simulink model "motor_ctrl"  (R2021a)
settings: configuration reference "f2_ctrl_config" (kept outside this file)
settings Model: DataDictionary=motor_data.sldd  Creator=Litao  LastModifiedBy=Litao
settings ConfigSetRef: SourceName=f2_ctrl_config

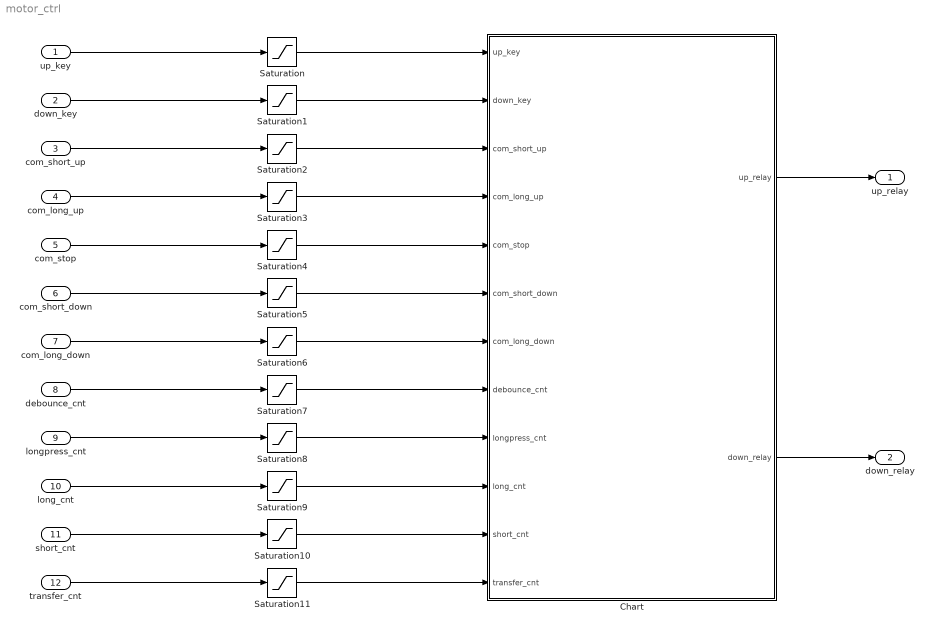
== system motor_ctrl ==
  up_key : Inport  OutDataTypeStr=int16
  down_key : Inport  Port=2  OutDataTypeStr=int16
  com_short_up : Inport  Port=3  OutDataTypeStr=int16
  com_long_up : Inport  Port=4  OutDataTypeStr=int16
  com_stop : Inport  Port=5  OutDataTypeStr=int16
  com_short_down : Inport  Port=6  OutDataTypeStr=int16
  com_long_down : Inport  Port=7  OutDataTypeStr=int16
  debounce_cnt : Inport  Port=8  OutDataTypeStr=int16
  longpress_cnt : Inport  Port=9  OutDataTypeStr=int16
  long_cnt : Inport  Port=10  OutDataTypeStr=int16
  short_cnt : Inport  Port=11  OutDataTypeStr=int16
  transfer_cnt : Inport  Port=12  OutDataTypeStr=int16
  Chart : Stateflow chart  TreatAsAtomicUnit=on
      settings: PortSchema="{\"entries\":[{\"content\":{\"sides\":[{\"content\":{\"connectorIds\":[\"In1\",\"In6\",\"In2\",\"In3\",\"In4\",\"In5\",\"In7\",\"In8\",\"In9\",\"In10\",\"In11\",\"In12\"]},\"type\":\"ConnectorPlacement.EquallySpacedRectSide\",\"uuid\":\"4c20fa99-1adf-4f22-ae93-c6186f058e35\"},{\"content\":{\"connectorIds\":[\"Out1\",\"Out2\"],\"side\":\"RIGHT\"},\"type\":\"ConnectorPlacement.EquallySpacedRectSide\",\"uuid\":\"7e4b4d75-813d-4fac-a5e7-b1188569f7b1\"},{\"content\":{\"connectorIds\":[],\"side\":\"TOP\"},\"type\":\"ConnectorPlacement.EquallySpacedRectSide\",\"uuid\":\"dfb94294-383a-4a0d-9cf2-9ac7874d8458\"}]},\"type\":\"ConnectorPlacement.EquallySpacedConnector\",\"uuid\":\"7d129faa-0032-4342-99de-de2067696b6a\"}],\"packageUris\":[\"http://schema.mathworks.com/mf0/Connector/R2020b\"],\"version\":\"1.0\"}"
  Saturation{,1..6} (7 alike) : Saturate  UpperLimit=1  LowerLimit=0
  Saturation10 : Saturate  UpperLimit=50  LowerLimit=20
  Saturation11 : Saturate  UpperLimit=50  LowerLimit=20
  Saturation7 : Saturate  UpperLimit=4  LowerLimit=1
  Saturation8 : Saturate  UpperLimit=200  LowerLimit=50
  Saturation9 : Saturate  UpperLimit=6000  LowerLimit=1000
  up_relay : Outport  OutDataTypeStr=int16
  down_relay : Outport  Port=2  OutDataTypeStr=int16
  wires:
  up_key/1 -> Saturation/1
  down_key/1 -> Saturation1/1
  com_short_up/1 -> Saturation2/1
  com_long_up/1 -> Saturation3/1
  com_stop/1 -> Saturation4/1
  com_short_down/1 -> Saturation5/1
  com_long_down/1 -> Saturation6/1
  Chart/1(up_relay) -> up_relay/1
  Chart/2(down_relay) -> down_relay/1
  debounce_cnt/1 -> Saturation7/1
  longpress_cnt/1 -> Saturation8/1
  long_cnt/1 -> Saturation9/1
  short_cnt/1 -> Saturation10/1
  transfer_cnt/1 -> Saturation11/1
  Saturation/1 -> Chart/1(up_key)
  Saturation1/1 -> Chart/6(down_key)
  Saturation2/1 -> Chart/2(com_short_up)
  Saturation3/1 -> Chart/3(com_long_up)
  Saturation4/1 -> Chart/4(com_stop)
  Saturation5/1 -> Chart/5(com_short_down)
  Saturation6/1 -> Chart/7(com_long_down)
  Saturation7/1 -> Chart/8(debounce_cnt)
  Saturation8/1 -> Chart/9(longpress_cnt)
  Saturation9/1 -> Chart/10(long_cnt)
  Saturation10/1 -> Chart/11(short_cnt)
  Saturation11/1 -> Chart/12(transfer_cnt)

== stateflow chart motor_ctrl/Chart ==
  state MOTOR_CTRL
    state COM_CMD [parallel]
      settings: executionOrder=1
      state SHORT_DOWN
        en: send(short_down_event,MOTOR)
      state IDLE
      state SHORT_UP
        en: send(short_up_event,MOTOR)
      state LONG_DOWN
        en: send(long_down_event,MOTOR)
      state LONG_UP
        en: send(long_up_event,MOTOR)
      state STOP
        en: send(stop_event,MOTOR)
      (default) -> MOTOR_CTRL.COM_CMD.IDLE
      MOTOR_CTRL.COM_CMD.IDLE -> MOTOR_CTRL.COM_CMD.SHORT_UP [order 3] : [com_short_up==1]
      MOTOR_CTRL.COM_CMD.IDLE -> MOTOR_CTRL.COM_CMD.SHORT_DOWN [order 5] : [com_short_down==1]
      MOTOR_CTRL.COM_CMD.SHORT_DOWN -> MOTOR_CTRL.COM_CMD.IDLE : [after(short_cnt,tick)]
      MOTOR_CTRL.COM_CMD.SHORT_UP -> MOTOR_CTRL.COM_CMD.IDLE : [after(short_cnt,tick)]
      MOTOR_CTRL.COM_CMD.IDLE -> MOTOR_CTRL.COM_CMD.LONG_DOWN [order 1] : [com_long_down==1]
      MOTOR_CTRL.COM_CMD.LONG_DOWN -> MOTOR_CTRL.COM_CMD.IDLE : [after(short_cnt,tick)]
      MOTOR_CTRL.COM_CMD.IDLE -> STOP [order 2] : [com_stop==1]
      STOP -> MOTOR_CTRL.COM_CMD.IDLE : [after(short_cnt,tick)]
      MOTOR_CTRL.COM_CMD.LONG_UP -> MOTOR_CTRL.COM_CMD.IDLE : [after(short_cnt,tick)]
      MOTOR_CTRL.COM_CMD.IDLE -> MOTOR_CTRL.COM_CMD.LONG_UP [order 4] : [com_long_up==1]
    state KEY_CMD [parallel]
      settings: executionOrder=2
      state DOWN_KEY_PRESSED
        state DOWN_CLICK
        state DOWN_DEBOUNCE
        state DOWN_LONGPRESS
          en: send(down_key_long_press,MOTOR)
        (default) -> DOWN_DEBOUNCE
        DOWN_DEBOUNCE -> DOWN_CLICK [order 1] : [after(debounce_cnt,tick)]
        DOWN_CLICK -> DOWN_LONGPRESS [order 2] : [after(longpress_cnt,tick)]
      state IDLE
      state UP_KEY_PRESSED
        state UP_DEBOUNCE
        state UP_CLICK
        state UP_LONGPRESS
          en: send(up_key_long_press,MOTOR)
        (default) -> UP_DEBOUNCE
        UP_DEBOUNCE -> UP_CLICK [order 1] : [after(debounce_cnt,tick)]
        UP_CLICK -> UP_LONGPRESS [order 2] : [after(longpress_cnt,tick)]
      (default) -> MOTOR_CTRL.KEY_CMD.IDLE
      MOTOR_CTRL.KEY_CMD.IDLE -> UP_KEY_PRESSED [order 1] : [up_key==1]
      MOTOR_CTRL.KEY_CMD.IDLE -> DOWN_DEBOUNCE [order 2] : [down_key==1]
      UP_DEBOUNCE -> MOTOR_CTRL.KEY_CMD.IDLE [order 2] : [up_key~=1]
      DOWN_DEBOUNCE -> MOTOR_CTRL.KEY_CMD.IDLE [order 2] : [down_key~=1]
      UP_CLICK -> MOTOR_CTRL.KEY_CMD.IDLE [order 1] : [up_key~=1]{send(up_key_click,MOTOR)}
      DOWN_CLICK -> MOTOR_CTRL.KEY_CMD.IDLE [order 1] : [down_key~=1]{send(down_key_click, MOTOR)}
      UP_LONGPRESS -> MOTOR_CTRL.KEY_CMD.IDLE : [up_key~=1]
      DOWN_LONGPRESS -> MOTOR_CTRL.KEY_CMD.IDLE : [down_key~=1]
    state MOTOR [parallel]
      settings: executionOrder=3
      state SHORT_DOWN
        en: down_relay=1;
        ex: down_relay=0;
      state OFF
      state SHORT_UP
        en: up_relay=1;
        ex: up_relay=0;
      state LONG_DOWN
        en: down_relay=1;
        ex: down_relay=0;
      state LONG_UP
        en: up_relay=1;
        ex: up_relay=0;
      state UP_TO_LONGDOWN
      state DOWN_TO_LONGUP
      (default) -> OFF
      OFF -> MOTOR_CTRL.MOTOR.SHORT_DOWN [order 3] : [down_key_click || short_down_event]
      OFF -> MOTOR_CTRL.MOTOR.SHORT_UP [order 1] : [up_key_click || short_up_event]
      MOTOR_CTRL.MOTOR.SHORT_UP -> OFF : [after(short_cnt,tick)]
      MOTOR_CTRL.MOTOR.SHORT_DOWN -> OFF : [after(short_cnt,tick)]
      OFF -> MOTOR_CTRL.MOTOR.LONG_UP [order 2] : [up_key_long_press || long_up_event]
      OFF -> MOTOR_CTRL.MOTOR.LONG_DOWN [order 4] : [down_key_long_press || long_down_event]
      MOTOR_CTRL.MOTOR.LONG_UP -> OFF [order 2] : [up_key_click || down_key_click ||stop_event ||after(long_cnt,tick)]
      MOTOR_CTRL.MOTOR.LONG_DOWN -> OFF [order 1] : [down_key_click || up_key_click || stop_event ||after(long_cnt,tick)]
      UP_TO_LONGDOWN -> MOTOR_CTRL.MOTOR.LONG_DOWN : [after(transfer_cnt, tick)]
      MOTOR_CTRL.MOTOR.LONG_UP -> UP_TO_LONGDOWN [order 1] : [down_key_long_press || long_down_event]
      MOTOR_CTRL.MOTOR.LONG_DOWN -> DOWN_TO_LONGUP [order 2] : [up_key_long_press || long_up_event]
      DOWN_TO_LONGUP -> MOTOR_CTRL.MOTOR.LONG_UP : [after(transfer_cnt, tick)]
  (default) -> MOTOR_CTRL
  data: up_key input; com_short_up input; com_long_up input; com_stop input; com_short_down input; down_key input; com_long_down input; up_relay output int16; down_relay output int16; debounce_cnt input; longpress_cnt input; long_cnt input; short_cnt input; transfer_cnt input
  events: long_down_event local FUNCTION_CALL_EVENT; long_up_event local FUNCTION_CALL_EVENT; short_down_event local FUNCTION_CALL_EVENT; short_up_event local FUNCTION_CALL_EVENT; stop_event local FUNCTION_CALL_EVENT; down_key_click local FUNCTION_CALL_EVENT; down_key_long_press local FUNCTION_CALL_EVENT; up_key_click local FUNCTION_CALL_EVENT; up_key_long_press local FUNCTION_CALL_EVENT
